simulink model "DT_Model_Matching_Desired"  (R2015a)
settings: Solver=FixedStepDiscrete  StartTime=0.0  StopTime=Tf  FixedStep=Ts  MaxStep=1e-5  RelTol=1e-4
values from neighbouring files (symbols this model uses):
  Ts = 0.05    [wheel_parameters.m]
undefined symbols (not defined in the file or in its folder): den_Go, num_Go
settings Model: Creator=throne  LastModifiedBy=throne
settings DataIOCC: SignalLoggingSaveFormat=ModelDataLogs  SignalLoggingName=sigsOut
settings OptimizationCC: ExpressionDepthLimit=2147483647
settings DebuggingCC: SaveWithParameterizedLinksMsg=none  UnderspecifiedInitializationDetection=Classic  MergeDetectMultiDrivingBlocksExec=none  SignalResolutionControl=TryResolveAllWithWarning  MultiTaskDSMMsg=warning  MultiTaskCondExecSysMsg=none  StateNameClashWarn=warning
settings HardwareCC: TargetUnknown=on
settings GRTTargetCC: CombineOutputUpdateFcns=off  GRTInterface=on

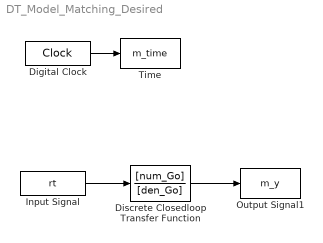
== system DT_Model_Matching_Desired ==
  Digital Clock : DigitalClock  SampleTime=Ts
  Discrete Closedloop Transfer Function : DiscreteTransferFcn  Numerator=[num_Go]  Denominator=[den_Go]  SampleTime=Ts
  "Input Signal " : FromWorkspace  VariableName=rt  SampleTime=Ts
  Output Signal1 : ToWorkspace  VariableName=m_y  SampleTime=-1
  Time : ToWorkspace  VariableName=m_time  SampleTime=-1
  wires:
  Digital Clock/1 -> Time/1
  Discrete Closedloop Transfer Function/1 -> Output Signal1/1
  "Input Signal "/1 -> Discrete Closedloop Transfer Function/1
